simulink model "OLD_SS_PID_Control_model"  (R2023a)
settings: Solver=FixedStepAuto  StartTime=0.0  StopTime=100  FixedStep=0.001  RelTol=1e-3
values from neighbouring files (symbols this model uses):
  A = [0 1;-k/m -c/m]    [SS_PID_Control.m]
  amp = 0.0005    [SS_PID_Control.m]
  B = [0;k_f/m]    [SS_PID_Control.m]
  C = [1 0]    [SS_PID_Control.m]
  D = 0    [SS_PID_Control.m]
  E = [0 0;c/m k/m]    [SS_PID_Control.m]
  fre = 300    [SS_PID_Control.m]
  Kd = 00070    (= 70)    [SS_PID_Control.m]
  Ki = 13000    [SS_PID_Control.m]
  Kp = 27000    [SS_PID_Control.m]
libraries: slpidlib x2
settings Model: Creator=z'k'x  LastModifiedBy=z'k'x

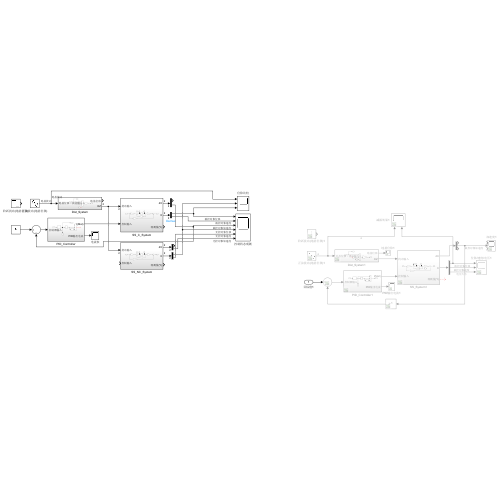
[thumbnail: Simulink's stored preview of the top-level diagram]
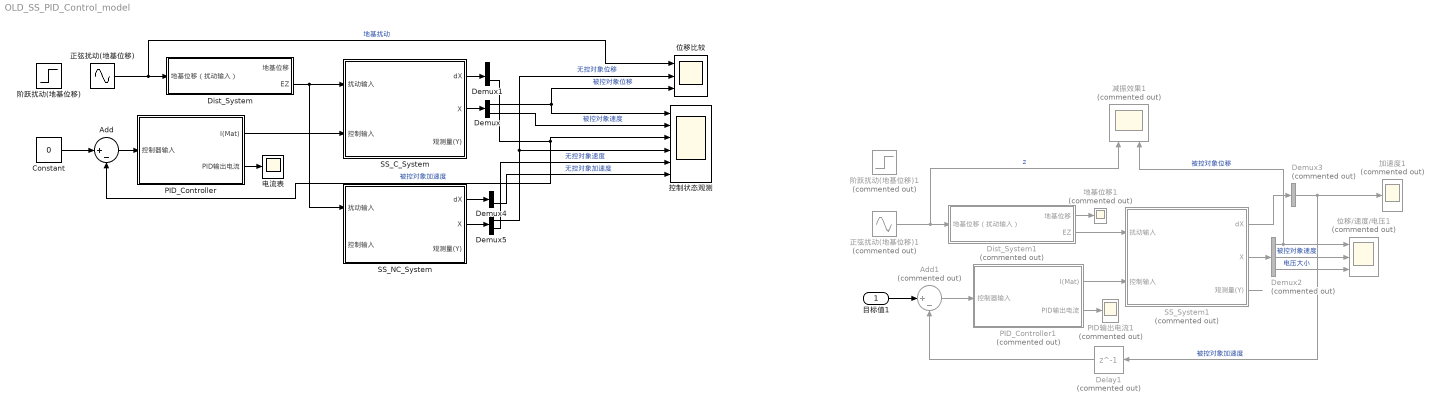
== system OLD_SS_PID_Control_model ==
  目标值1 : Inport
  Add : Sum  Inputs=|+-
  Add1 : Sum  Commented=on  Inputs=|+-
  Constant : Constant  Value=0
  Delay1 : Delay  Commented=on  DelayLength=1  InitialCondition=0
  Demux{,1,4..5} (4 alike) : Demux  Outputs=2
  Demux2 : Demux  Commented=on  Outputs=3
  Demux3 : Demux  Commented=on  Outputs=3
  Dist_System : Subsystem
  Dist_System1 : Subsystem  Commented=on
  PID_Controller : Subsystem
  PID_Controller1 : Subsystem  Commented=on
  PID输出电流1 : Scope  Commented=on
  SS_C_System : Subsystem
  SS_NC_System : Subsystem
  SS_System1 : Subsystem  Commented=on
  位移/速度/电压1 : Scope  Commented=on  NumInputPorts=3
  位移比较 : Scope  NumInputPorts=3
  减振效果1 : Scope  Commented=on  NumInputPorts=2
  加速度1 : Scope  Commented=on  NumInputPorts=3
  地基位移1 : Scope  Commented=on
  控制状态观测 : Scope  NumInputPorts=6
  正弦扰动(地基位移) : Sin  Amplitude=amp  Frequency=fre  SampleTime=0
  正弦扰动(地基位移)1 : Sin  Commented=on  Amplitude=amp  Frequency=17.38*pi  SampleTime=0
  电流表 : Scope
  阶跃扰动(地基位移) : Step  Time=0.1  Before=0.01  After=0  SampleTime=0
  阶跃扰动(地基位移)1 : Step  Commented=on  Time=0.1  Before=0.01  After=0  SampleTime=0
  wires:
  Constant/1 -> Add/1
  Demux/2 -> 控制状态观测/2  "被控对象速度"
  Demux/1 -> 位移比较/3, 控制状态观测/1  "被控对象位移"
  Add/1 -> PID_Controller/1(控制器输入)
  PID_Controller/2(PID输出电流) -> 电流表/1
  正弦扰动(地基位移)/1 -> 位移比较/1, Dist_System/1(地基位移（扰动输入）)  "地基扰动"
  Dist_System/2(EZ) -> SS_C_System/1(扰动输入), SS_NC_System/1(扰动输入)
  SS_C_System/2(X) -> Demux/1
  Demux1/2 -> 控制状态观测/3, Add/2  "被控对象加速度"
  SS_C_System/1(dX) -> Demux1/1
  PID_Controller/1(I(Mat)) -> SS_C_System/2(控制输入)
  正弦扰动(地基位移)1/1 -> 减振效果1/1, Dist_System1/1(地基位移（扰动输入）)  "z"
  PID_Controller1/1(I(Mat)) -> SS_System1/2(控制输入)
  Dist_System1/2(EZ) -> SS_System1/1(扰动输入)
  SS_System1/1(dX) -> Demux3/1
  Demux2/1 -> 位移/速度/电压1/1, 减振效果1/2  "被控对象位移"
  Demux2/2 -> 位移/速度/电压1/2  "被控对象速度"
  PID_Controller1/2(PID输出电流) -> PID输出电流1/1
  SS_System1/2(X) -> Demux2/1
  Dist_System1/1(地基位移) -> 地基位移1/1
  Add1/1 -> PID_Controller1/1(控制器输入)
  SS_System1/3(观测量(Y)) -> ?
  Demux3/2 -> Delay1/1, 加速度1/2  "被控对象加速度"
  Demux2/3 -> 位移/速度/电压1/3  "电压大小"
  目标值1/1 -> Add1/1
  Delay1/1 -> Add1/2
  SS_NC_System/1(dX) -> Demux4/1
  Demux4/2 -> 控制状态观测/6  "无控对象加速度"
  SS_NC_System/2(X) -> Demux5/1
  Demux5/1 -> 位移比较/2, 控制状态观测/4  "无控对象位移"
  Demux5/2 -> 控制状态观测/5  "无控对象速度"

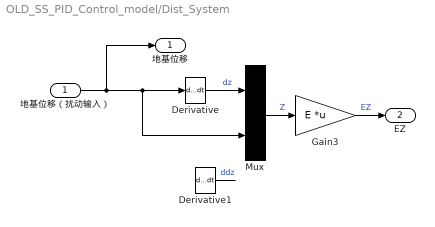
== system OLD_SS_PID_Control_model/Dist_System ==
  地基位移（扰动输入） : Inport
  Derivative : Derivative
  Derivative1 : Derivative
  Gain3 : Gain  Gain=E  Multiplication=Matrix(K*u) (u vector)
  Mux : Mux  Inputs=2
      settings: DisplayOption=signals
  地基位移 : Outport
  EZ : Outport  Port=2
  wires:
  Gain3/1 -> EZ/1  "EZ"
  Mux/1 -> Gain3/1  "Z"
  Derivative/1 -> Mux/1  "dz"
  Derivative1/1 -> ?  "ddz"
  地基位移（扰动输入）/1 -> 地基位移/1, Derivative/1, Mux/2

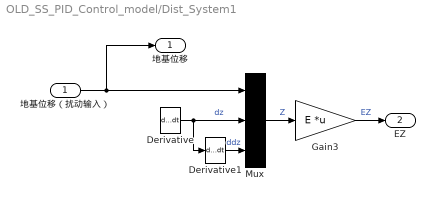
== system OLD_SS_PID_Control_model/Dist_System1 ==
  地基位移（扰动输入） : Inport
  Derivative : Derivative
  Derivative1 : Derivative
  Gain3 : Gain  Gain=E  Multiplication=Matrix(K*u) (u vector)
  Mux : Mux  Inputs=3
      settings: DisplayOption=signals
  地基位移 : Outport
  EZ : Outport  Port=2
  wires:
  Gain3/1 -> EZ/1  "EZ"
  地基位移（扰动输入）/1 -> 地基位移/1, Mux/1
  Mux/1 -> Gain3/1  "Z"
  Derivative/1 -> Mux/2, Derivative1/1  "dz"
  Derivative1/1 -> Mux/3  "ddz"
  ? -> Derivative/1

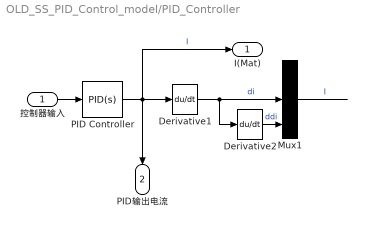
== system OLD_SS_PID_Control_model/PID_Controller ==
  控制器输入 : Inport
  Derivative1 : Derivative
  Derivative2 : Derivative
  Mux1 : Mux  Inputs=3
      settings: DisplayOption=signals
  PID Controller : slpidlib/PID Controller  Controller=PID  Form=Parallel  TimeDomain=Continuous-time  UseExternalTs=off  SampleTime=-1  IntegratorMethod=Forward Euler  FilterMethod=Forward Euler  ControllerParametersSource=internal  P=Kp  I=Ki  UseKiTs=off  D=Kd  N=100  UseFilter=on  TunerSelectOption=Transfer Function Based (PID Tuner App)  InitialConditionSource=internal  InitialConditionForIntegrator=0  InitialConditionForFilter=0  DifferentiatorICPrevScaledInput=0  ExternalReset=none  TrackingMode=off  Kt=1  LimitOutput=off  SatLimitsSource=internal  UpperSaturationLimit=inf  LowerSaturationLimit=-inf  LinearizeAsGain=on  AntiWindupMode=none  Kb=1  LimitIntegrator=off  UpperIntegratorSaturationLimit=inf  LowerIntegratorSaturationLimit=-inf  POutMin=[]  POutMax=[]  IOutMin=[]  IOutMax=[]  DOutMin=[]  DOutMax=[]  NOutMin=[]  NOutMax=[]  SumOutMin=[]  SumOutMax=[]  SaturationOutMin=[]  SaturationOutMax=[]  PParamMin=[]  PParamMax=[]  IParamMin=[]  IParamMax=[]  DParamMin=[]  DParamMax=[]  NParamMin=[]  NParamMax=[]  KbParamMin=[]  KbParamMax=[]  KtParamMin=[]  KtParamMax=[]  KbOutMin=[]  KbOutMax=[]  KtOutMin=[]  KtOutMax=[]  IntegratorOutMin=[]  IntegratorOutMax=[]  FilterOutMin=[]  FilterOutMax=[]  SumI1OutMin=[]  SumI1OutMax=[]  SumI2OutMin=[]  SumI2OutMax=[]  SumI3OutMin=[]  SumI3OutMax=[]  SumI4OutMin=[]  SumI4OutMax=[]  SumDOutMin=[]  SumDOutMax=[]  DifferentiatorOutMin=[]  DifferentiatorOutMax=[]  FilterDiffOutCoefMin=[]  FilterDiffOutCoefMax=[]  ReciprocalOutMin=[]  ReciprocalOutMax=[]  SumDenOutMin=[]  SumDenOutMax=[]  SumNumOutMin=[]  SumNumOutMax=[]  DivideOutMin=[]  DivideOutMax=[]  UdiffTsProdOutMin=[]  UdiffTsProdOutMax=[]  NTsProdOutMin=[]  NTsProdOutMax=[]  UintegralTsProdOutMin=[]  UintegralTsProdOutMax=[]  UngainTsProdOutMin=[]  UngainTsProdOutMax=[]  ClampingZeroOutDataTypeStr=Inherit: Inherit via back propagation  ClampingZeroOutMin=[]  ClampingZeroOutMax=[]  FilterDenConstantOutDataTypeStr=Inherit: Inherit via back propagation  FilterDenConstantOutMin=[]  FilterDenConstantOutMax=[]  PCopyOutDataTypeStr=Inherit: Inherit via back propagation  PCopyOutMin=[]  PCopyOutMax=[]  NCopyOutDataTypeStr=Inherit: Inherit via back propagation  NCopyOutMin=[]  NCopyOutMax=[]  IntegratorContinuousStateAttributes=''  IntegratorStateMustResolveToSignalObject=off  IntegratorRTWStateStorageClass=Auto  FilterContinuousStateAttributes=''  FilterStateMustResolveToSignalObject=off  FilterRTWStateStorageClass=Auto  ParallelPVariant=InternalParameters  IdealPVariant=Disabled  IVariant=InternalParameters  DVariant=InternalParameters  IntegratorVariant=Continuous  SatVariant=Disabled  AWVariant=Passthrough  PCopyVariant=Disabled  TRVariant=Disabled  FdbkBlocksVariant=Forward  IdealPFdbkVariant=Disabled  SatFdbkVariant=Disabled  DerivativeFilterVariant=ContFilter  NVariant=InternalParameters  NCopyVariant=Disabled  FilterICVariant=InternalICsFilter  IntegratorICVariant=InternalICs  ExternalResetVariant=Disabled  TRSumVariant=Passthrough  SumFdbkVariant=Disabled  SumVariant=Sum_PID  TsampFilterVariant=InternalTs  TsampNgainVariant=Passthrough  TsampIntegralVariant=Disabled_SignalSpec  ExternalSaturationOutDataTypeStr=Inherit: Same as second input
  I(Mat) : Outport
  PID输出电流 : Outport  Port=2
  wires:
  PID Controller/1 -> I(Mat)/1, PID输出电流/1, Derivative1/1  "I"
  Derivative1/1 -> Derivative2/1, Mux1/2  "di"
  Derivative2/1 -> Mux1/3  "ddi"
  控制器输入/1 -> PID Controller/1
  Mux1/1 -> ?  "I"

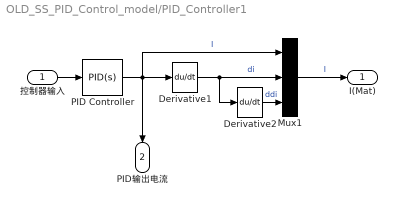
== system OLD_SS_PID_Control_model/PID_Controller1 ==
  控制器输入 : Inport
  Derivative1 : Derivative
  Derivative2 : Derivative
  Mux1 : Mux  Inputs=3
      settings: DisplayOption=signals
  PID Controller : slpidlib/PID Controller  Controller=PID  Form=Parallel  TimeDomain=Continuous-time  UseExternalTs=off  SampleTime=-1  IntegratorMethod=Forward Euler  FilterMethod=Forward Euler  ControllerParametersSource=internal  P=Kp  I=Ki  UseKiTs=off  D=Kd  N=100  UseFilter=on  TunerSelectOption=Transfer Function Based (PID Tuner App)  InitialConditionSource=internal  InitialConditionForIntegrator=0  InitialConditionForFilter=0  DifferentiatorICPrevScaledInput=0  ExternalReset=none  TrackingMode=off  Kt=1  LimitOutput=off  SatLimitsSource=internal  UpperSaturationLimit=inf  LowerSaturationLimit=-inf  LinearizeAsGain=on  AntiWindupMode=none  Kb=1  LimitIntegrator=off  UpperIntegratorSaturationLimit=inf  LowerIntegratorSaturationLimit=-inf  POutMin=[]  POutMax=[]  IOutMin=[]  IOutMax=[]  DOutMin=[]  DOutMax=[]  NOutMin=[]  NOutMax=[]  SumOutMin=[]  SumOutMax=[]  SaturationOutMin=[]  SaturationOutMax=[]  PParamMin=[]  PParamMax=[]  IParamMin=[]  IParamMax=[]  DParamMin=[]  DParamMax=[]  NParamMin=[]  NParamMax=[]  KbParamMin=[]  KbParamMax=[]  KtParamMin=[]  KtParamMax=[]  KbOutMin=[]  KbOutMax=[]  KtOutMin=[]  KtOutMax=[]  IntegratorOutMin=[]  IntegratorOutMax=[]  FilterOutMin=[]  FilterOutMax=[]  SumI1OutMin=[]  SumI1OutMax=[]  SumI2OutMin=[]  SumI2OutMax=[]  SumI3OutMin=[]  SumI3OutMax=[]  SumI4OutMin=[]  SumI4OutMax=[]  SumDOutMin=[]  SumDOutMax=[]  DifferentiatorOutMin=[]  DifferentiatorOutMax=[]  FilterDiffOutCoefMin=[]  FilterDiffOutCoefMax=[]  ReciprocalOutMin=[]  ReciprocalOutMax=[]  SumDenOutMin=[]  SumDenOutMax=[]  SumNumOutMin=[]  SumNumOutMax=[]  DivideOutMin=[]  DivideOutMax=[]  UdiffTsProdOutMin=[]  UdiffTsProdOutMax=[]  NTsProdOutMin=[]  NTsProdOutMax=[]  UintegralTsProdOutMin=[]  UintegralTsProdOutMax=[]  UngainTsProdOutMin=[]  UngainTsProdOutMax=[]  ClampingZeroOutDataTypeStr=Inherit: Inherit via back propagation  ClampingZeroOutMin=[]  ClampingZeroOutMax=[]  FilterDenConstantOutDataTypeStr=Inherit: Inherit via back propagation  FilterDenConstantOutMin=[]  FilterDenConstantOutMax=[]  PCopyOutDataTypeStr=Inherit: Inherit via back propagation  PCopyOutMin=[]  PCopyOutMax=[]  NCopyOutDataTypeStr=Inherit: Inherit via back propagation  NCopyOutMin=[]  NCopyOutMax=[]  IntegratorContinuousStateAttributes=''  IntegratorStateMustResolveToSignalObject=off  IntegratorRTWStateStorageClass=Auto  FilterContinuousStateAttributes=''  FilterStateMustResolveToSignalObject=off  FilterRTWStateStorageClass=Auto  ParallelPVariant=InternalParameters  IdealPVariant=Disabled  IVariant=InternalParameters  DVariant=InternalParameters  IntegratorVariant=Continuous  SatVariant=Disabled  AWVariant=Passthrough  PCopyVariant=Disabled  TRVariant=Disabled  FdbkBlocksVariant=Forward  IdealPFdbkVariant=Disabled  SatFdbkVariant=Disabled  DerivativeFilterVariant=ContFilter  NVariant=InternalParameters  NCopyVariant=Disabled  FilterICVariant=InternalICsFilter  IntegratorICVariant=InternalICs  ExternalResetVariant=Disabled  TRSumVariant=Passthrough  SumFdbkVariant=Disabled  SumVariant=Sum_PID  TsampFilterVariant=InternalTs  TsampNgainVariant=Passthrough  TsampIntegralVariant=Disabled_SignalSpec  ExternalSaturationOutDataTypeStr=Inherit: Same as second input
  I(Mat) : Outport
  PID输出电流 : Outport  Port=2
  wires:
  PID Controller/1 -> PID输出电流/1, Derivative1/1, Mux1/1  "I"
  Derivative1/1 -> Derivative2/1, Mux1/2  "di"
  Derivative2/1 -> Mux1/3  "ddi"
  控制器输入/1 -> PID Controller/1
  Mux1/1 -> I(Mat)/1  "I"

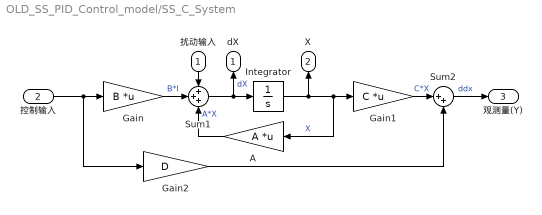
== system OLD_SS_PID_Control_model/SS_C_System ==
  扰动输入 : Inport
  控制输入 : Inport  Port=2
  A : Gain  Gain=A  Multiplication=Matrix(K*u) (u vector)
  Gain : Gain  Gain=B  Multiplication=Matrix(K*u) (u vector)
  Gain1 : Gain  Gain=C  Multiplication=Matrix(K*u) (u vector)
  Gain2 : Gain  Gain=D
  Integrator : Integrator
  Sum1 : Sum  Inputs=+++
  Sum2 : Sum  Inputs=|++
  dX : Outport
  X : Outport  Port=2
  观测量(Y) : Outport  Port=3
  wires:
  Gain2/1 -> Sum2/2
  Integrator/1 -> A/1, Gain1/1, X/1  "X"
  Sum1/1 -> dX/1, Integrator/1  "dX"
  Gain/1 -> Sum1/2  "B*I"
  Gain1/1 -> Sum2/1  "C*X"
  A/1 -> Sum1/3  "A*X"
  Sum2/1 -> 观测量(Y)/1  "ddx"
  控制输入/1 -> Gain2/1, Gain/1
  扰动输入/1 -> Sum1/1

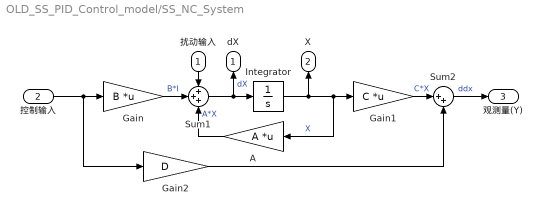
== system OLD_SS_PID_Control_model/SS_NC_System ==
  扰动输入 : Inport
  控制输入 : Inport  Port=2
  A : Gain  Gain=A  Multiplication=Matrix(K*u) (u vector)
  Gain : Gain  Gain=B  Multiplication=Matrix(K*u) (u vector)
  Gain1 : Gain  Gain=C  Multiplication=Matrix(K*u) (u vector)
  Gain2 : Gain  Gain=D
  Integrator : Integrator
  Sum1 : Sum  Inputs=+++
  Sum2 : Sum  Inputs=|++
  dX : Outport
  X : Outport  Port=2
  观测量(Y) : Outport  Port=3
  wires:
  Gain2/1 -> Sum2/2
  Integrator/1 -> A/1, Gain1/1, X/1  "X"
  Sum1/1 -> dX/1, Integrator/1  "dX"
  Gain/1 -> Sum1/2  "B*I"
  Gain1/1 -> Sum2/1  "C*X"
  A/1 -> Sum1/3  "A*X"
  Sum2/1 -> 观测量(Y)/1  "ddx"
  控制输入/1 -> Gain2/1, Gain/1
  扰动输入/1 -> Sum1/1

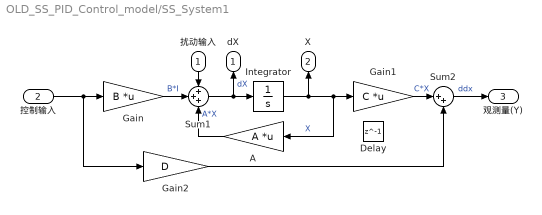
== system OLD_SS_PID_Control_model/SS_System1 ==
  扰动输入 : Inport
  控制输入 : Inport  Port=2
  A : Gain  Gain=A  Multiplication=Matrix(K*u) (u vector)
  Delay : Delay  DelayLength=1  InitialCondition=0
  Gain : Gain  Gain=B  Multiplication=Matrix(K*u) (u vector)
  Gain1 : Gain  Gain=C  Multiplication=Matrix(K*u) (u vector)
  Gain2 : Gain  Gain=D
  Integrator : Integrator
  Sum1 : Sum  Inputs=+++
  Sum2 : Sum  Inputs=|++
  dX : Outport
  X : Outport  Port=2
  观测量(Y) : Outport  Port=3
  wires:
  Gain2/1 -> Sum2/2
  Integrator/1 -> A/1, Gain1/1, X/1  "X"
  Sum1/1 -> dX/1, Integrator/1  "dX"
  Gain/1 -> Sum1/2  "B*I"
  Gain1/1 -> Sum2/1  "C*X"
  A/1 -> Sum1/3  "A*X"
  Sum2/1 -> 观测量(Y)/1  "ddx"
  控制输入/1 -> Gain2/1, Gain/1
  扰动输入/1 -> Sum1/1
